simulink model "CSTHLinearMOOPID"  (R2019b)
settings: Solver=VariableStepAuto  StartTime=0.0  StopTime=1000  RelTol=1e-3
values from neighbouring files (symbols this model uses):
  beta = MOOResults.beta    [TuningMOOToolCSTH.m]    (also in TuningMOOToolCSTH3Fun.m)
  K = 0.3658    [TuningCSTH.m]    (also in TuningMOOCSTH.m; TuningMOOToolCSTH.m)
  Kp = MOOResults.Kp    [TuningMOOToolCSTH.m]    (also in TuningMOOToolCSTH3Fun.m)
  L = 24.736    [TuningCSTH.m]    (also in TuningMOOCSTH.m; TuningMOOToolCSTH.m)
  T1 = 52.861    [TuningCSTH.m]    (also in TuningMOOCSTH.m; TuningMOOToolCSTH.m)
  T2 = 52.805    [TuningCSTH.m]    (also in TuningMOOCSTH.m; TuningMOOToolCSTH.m)
  Td = MOOResults.Td    [TuningMOOToolCSTH.m]    (also in TuningMOOToolCSTH3Fun.m)
  Ti = MOOResults.Ti    [TuningMOOToolCSTH.m]    (also in TuningMOOToolCSTH3Fun.m)
libraries: simulink x2
settings Model: Creator=david  LastModifiedBy=david

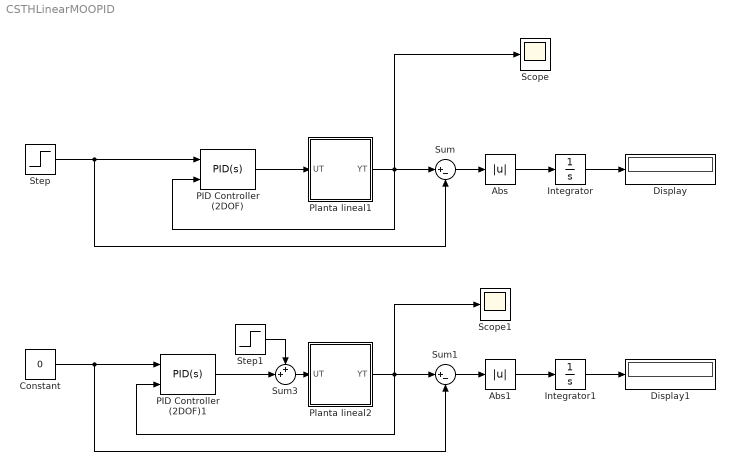
== system CSTHLinearMOOPID ==
  Abs : Abs
  Abs1 : Abs
  Constant : Constant  Value=0
  Display : Display
  Display1 : Display
  Integrator : Integrator
  Integrator1 : Integrator
  PID Controller (2DOF) : simulink/Continuous/PID Controller (2DOF)  Controller=PID  Form=Ideal  TimeDomain=Continuous-time  SampleTime=-1  IntegratorMethod=Forward Euler  FilterMethod=Forward Euler  ControllerParametersSource=internal  P=Kp  I=1/Ti  D=Td  UseFilter=on  N=100  b=beta  c=0  TunerSelectOption=Transfer Function Based (PID Tuner App)  InitialConditionSource=internal  InitialConditionForIntegrator=0  InitialConditionForFilter=0  DifferentiatorICPrevScaledInput=0  ExternalReset=none  TrackingMode=off  Kt=1  LimitOutput=off  UpperSaturationLimit=inf  LowerSaturationLimit=-inf  LinearizeAsGain=on  AntiWindupMode=none  Kb=1  POutMin=[]  POutMax=[]  IOutMin=[]  IOutMax=[]  DOutMin=[]  DOutMax=[]  NOutMin=[]  NOutMax=[]  bOutMin=[]  bOutMax=[]  cOutMin=[]  cOutMax=[]  SumOutMin=[]  SumOutMax=[]  SaturationOutMin=[]  SaturationOutMax=[]  PParamMin=[]  PParamMax=[]  IParamMin=[]  IParamMax=[]  DParamMin=[]  DParamMax=[]  NParamMin=[]  NParamMax=[]  bParamMin=[]  bParamMax=[]  cParamMin=[]  cParamMax=[]  KbParamMin=[]  KbParamMax=[]  KtParamMin=[]  KtParamMax=[]  KbOutMin=[]  KbOutMax=[]  KtOutMin=[]  KtOutMax=[]  IntegratorOutMin=[]  IntegratorOutMax=[]  FilterOutMin=[]  FilterOutMax=[]  SumI1OutMin=[]  SumI1OutMax=[]  SumI2OutMin=[]  SumI2OutMax=[]  SumI3OutMin=[]  SumI3OutMax=[]  SumI4OutMin=[]  SumI4OutMax=[]  SumDOutMin=[]  SumDOutMax=[]  Sum1OutMin=[]  Sum1OutMax=[]  Sum2OutMin=[]  Sum2OutMax=[]  Sum3OutMin=[]  Sum3OutMax=[]  DifferentiatorOutMin=[]  DifferentiatorOutMax=[]  FilterDiffOutCoefMin=[]  FilterDiffOutCoefMax=[]  ReciprocalOutMin=[]  ReciprocalOutMax=[]  SumDenOutMin=[]  SumDenOutMax=[]  SumNumOutMin=[]  SumNumOutMax=[]  DivideOutMin=[]  DivideOutMax=[]  IntegratorContinuousStateAttributes=''  IntegratorStateMustResolveToSignalObject=off  IntegratorRTWStateStorageClass=Auto  FilterContinuousStateAttributes=''  FilterStateMustResolveToSignalObject=off  FilterRTWStateStorageClass=Auto  ParallelPVariant=Passthrough  IdealPVariant=InternalParameters  IVariant=InternalParameters  DVariant=InternalParameters  bVariant=InternalParameters  cVariant=InternalParameters  IntegratorVariant=Continuous  SatVariant=Disabled  AWVariant=Passthrough  PCopyVariant=Disabled  TRVariant=Disabled  FdbkBlocksVariant=Forward  IdealPFdbkVariant=Disabled  SatFdbkVariant=Disabled  DerivativeFilterVariant=ContFilter  NVariant=InternalParameters  NCopyVariant=Disabled  FilterICVariant=InternalICsFilter  IntegratorICVariant=InternalICs  ExternalResetVariant=Disabled  TRSumVariant=Passthrough  SumFdbkVariant=Disabled  SumVariant=Sum_PID
  PID Controller (2DOF)1 : simulink/Continuous/PID Controller (2DOF)  Controller=PID  Form=Ideal  TimeDomain=Continuous-time  SampleTime=-1  IntegratorMethod=Forward Euler  FilterMethod=Forward Euler  ControllerParametersSource=internal  P=Kp  I=1/Ti  D=Td  UseFilter=on  N=100  b=beta  c=0  TunerSelectOption=Transfer Function Based (PID Tuner App)  InitialConditionSource=internal  InitialConditionForIntegrator=0  InitialConditionForFilter=0  DifferentiatorICPrevScaledInput=0  ExternalReset=none  TrackingMode=off  Kt=1  LimitOutput=off  UpperSaturationLimit=inf  LowerSaturationLimit=-inf  LinearizeAsGain=on  AntiWindupMode=none  Kb=1  POutMin=[]  POutMax=[]  IOutMin=[]  IOutMax=[]  DOutMin=[]  DOutMax=[]  NOutMin=[]  NOutMax=[]  bOutMin=[]  bOutMax=[]  cOutMin=[]  cOutMax=[]  SumOutMin=[]  SumOutMax=[]  SaturationOutMin=[]  SaturationOutMax=[]  PParamMin=[]  PParamMax=[]  IParamMin=[]  IParamMax=[]  DParamMin=[]  DParamMax=[]  NParamMin=[]  NParamMax=[]  bParamMin=[]  bParamMax=[]  cParamMin=[]  cParamMax=[]  KbParamMin=[]  KbParamMax=[]  KtParamMin=[]  KtParamMax=[]  KbOutMin=[]  KbOutMax=[]  KtOutMin=[]  KtOutMax=[]  IntegratorOutMin=[]  IntegratorOutMax=[]  FilterOutMin=[]  FilterOutMax=[]  SumI1OutMin=[]  SumI1OutMax=[]  SumI2OutMin=[]  SumI2OutMax=[]  SumI3OutMin=[]  SumI3OutMax=[]  SumI4OutMin=[]  SumI4OutMax=[]  SumDOutMin=[]  SumDOutMax=[]  Sum1OutMin=[]  Sum1OutMax=[]  Sum2OutMin=[]  Sum2OutMax=[]  Sum3OutMin=[]  Sum3OutMax=[]  DifferentiatorOutMin=[]  DifferentiatorOutMax=[]  FilterDiffOutCoefMin=[]  FilterDiffOutCoefMax=[]  ReciprocalOutMin=[]  ReciprocalOutMax=[]  SumDenOutMin=[]  SumDenOutMax=[]  SumNumOutMin=[]  SumNumOutMax=[]  DivideOutMin=[]  DivideOutMax=[]  IntegratorContinuousStateAttributes=''  IntegratorStateMustResolveToSignalObject=off  IntegratorRTWStateStorageClass=Auto  FilterContinuousStateAttributes=''  FilterStateMustResolveToSignalObject=off  FilterRTWStateStorageClass=Auto  ParallelPVariant=Passthrough  IdealPVariant=InternalParameters  IVariant=InternalParameters  DVariant=InternalParameters  bVariant=InternalParameters  cVariant=InternalParameters  IntegratorVariant=Continuous  SatVariant=Disabled  AWVariant=Passthrough  PCopyVariant=Disabled  TRVariant=Disabled  FdbkBlocksVariant=Forward  IdealPFdbkVariant=Disabled  SatFdbkVariant=Disabled  DerivativeFilterVariant=ContFilter  NVariant=InternalParameters  NCopyVariant=Disabled  FilterICVariant=InternalICsFilter  IntegratorICVariant=InternalICs  ExternalResetVariant=Disabled  TRSumVariant=Passthrough  SumFdbkVariant=Disabled  SumVariant=Sum_PID
  Planta lineal1 : Subsystem
  Planta lineal2 : Subsystem
  Scope : Scope
  Scope1 : Scope
  Step : Step  Time=0  SampleTime=0
  Step1 : Step  Time=0  SampleTime=0
  Sum : Sum  Inputs=|+-
  Sum1 : Sum  Inputs=|+-
  Sum3 : Sum  Inputs=++|
  wires:
  Planta lineal1/1(YT) -> Scope/1, PID Controller (2DOF)/2, Sum/1
  Step/1 -> Sum/2, PID Controller (2DOF)/1
  PID Controller (2DOF)/1 -> Planta lineal1/1(UT)
  Constant/1 -> Sum1/2, PID Controller (2DOF)1/1
  Step1/1 -> Sum3/1
  Planta lineal2/1(YT) -> Scope1/1, PID Controller (2DOF)1/2, Sum1/1
  Sum3/1 -> Planta lineal2/1(UT)
  Sum/1 -> Abs/1
  Abs/1 -> Integrator/1
  Integrator/1 -> Display/1
  Sum1/1 -> Abs1/1
  Abs1/1 -> Integrator1/1
  Integrator1/1 -> Display1/1
  PID Controller (2DOF)1/1 -> Sum3/2

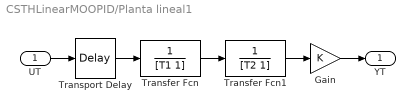
== system CSTHLinearMOOPID/Planta lineal1 ==
  UT : Inport
  Gain : Gain  Gain=K
  Transfer Fcn : TransferFcn  Denominator=[T1 1]
  Transfer Fcn1 : TransferFcn  Denominator=[T2 1]
  Transport Delay : TransportDelay  DelayTime=L  BufferSize=4096
  YT : Outport
  wires:
  Transfer Fcn1/1 -> Gain/1
  Transport Delay/1 -> Transfer Fcn/1
  Transfer Fcn/1 -> Transfer Fcn1/1
  UT/1 -> Transport Delay/1
  Gain/1 -> YT/1

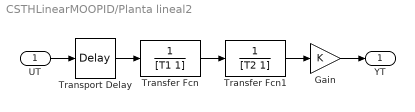
== system CSTHLinearMOOPID/Planta lineal2 ==
  UT : Inport
  Gain : Gain  Gain=K
  Transfer Fcn : TransferFcn  Denominator=[T1 1]
  Transfer Fcn1 : TransferFcn  Denominator=[T2 1]
  Transport Delay : TransportDelay  DelayTime=L  BufferSize=4096
  YT : Outport
  wires:
  Transfer Fcn1/1 -> Gain/1
  Transport Delay/1 -> Transfer Fcn/1
  Transfer Fcn/1 -> Transfer Fcn1/1
  UT/1 -> Transport Delay/1
  Gain/1 -> YT/1
